simulink model "hcu_main_ADASwEPS"  (Simulink 8.2)
settings: Solver=FixedStepDiscrete  StartTime=0.0  StopTime=inf  FixedStep=0.001  RelTol=1e-3
PostLoadFcn:
  | , if any(exist('dsrtsu_mdlpostloadfcn', 'file') == [2, 3, 6]), try dsrtsu_mdlpostloadfcn('Execute', bdroot); catch fprintf('Error in PostLoadFcn (dsrtsu_mdlpostloadfcn) for model "%s":\n %s\n', bdroot, lasterr); end, end,
values from neighbouring files (symbols this model uses):
  C_TASK_1MS_S = (	C_TICK_TIME_S       )    [hcu_local_hdr.m]    (also in temp_ovrd_values.m = double(	0.001                  ))
  C_TICK_TIME_S = single(	0.005	    	)    [hcu_local_hdr.m]
  ENUM_EPSLFCSTATUS_ACTIVE = uint8(  2  )    [hcu_local_hdr.m]
  ENUM_EPSLFCSTATUS_TRANSITION = uint8(  3  )    [hcu_local_hdr.m]
  ENUM_EPSLKASTATUS_ACTIVE = uint8(  2  )    [hcu_local_hdr.m]
  ENUM_EPSMODEREQ_ANGLE = uint8(  1  )    [hcu_local_hdr.m]
  ENUM_EPSMODEREQ_INTERNAL = uint8(  0  )    [hcu_local_hdr.m]
  ENUM_EPSMODEREQ_TORQUE = uint8(  2  )    [hcu_local_hdr.m]
  ENUM_GEARPOSN_1ST = uint8(  1  )    [hcu_local_hdr.m]
  ENUM_GEARPOSN_2ND = uint8(  2  )    [hcu_local_hdr.m]
  ENUM_GEARPOSN_3RD = uint8(  3  )    [hcu_local_hdr.m]
  ENUM_GEARPOSN_4TH = uint8(  4  )    [hcu_local_hdr.m]
  ENUM_GEARPOSN_5TH = uint8(  5  )    [hcu_local_hdr.m]
  ENUM_GEARPOSN_6TH = uint8(  6  )    [hcu_local_hdr.m]
  ENUM_GEARPOSN_R = uint8(  7  )    [hcu_local_hdr.m]
  FALSE = boolean( 0 )    [hcu_local_hdr.m]
  TRUE = boolean( 1 )    [hcu_local_hdr.m]
undefined symbols (not defined in the file or in its folder): AISP_EPSCurrent_pct, AISP_TqASensorDelta_pct, AISP_TqBSensorDelta_pct, dHAL_IN, hal, INVALID_ABS1_TIMEOUT, INVALID_ABS2_TIMEOUT, INVALID_ABS3_TIMEOUT, INVALID_ABS4_TIMEOUT, INVALID_AC1_TIMEOUT, INVALID_ADASTORQ_REQ, INVALID_BCM1_TIMEOUT, INVALID_BCM2_TIMEOUT, INVALID_BOOSTER_VAC, INVALID_CSW1_TIMEOUT, INVALID_CUR_VEHDECE, INVALID_CURBRAKEDECE_REQ, INVALID_CURSTEERANG_REQ, INVALID_CURSTEERTQ_REQ, INVALID_ECM1_TIMEOUT, INVALID_ECM2_TIMEOUT, INVALID_ECM3_TIMEOUT, INVALID_ECM9_TIMEOUT, INVALID_ENG_TORQUE_FRICTIONAL, INVALID_ENG_TORQUE_INDICATED, INVALID_ENG_TORQUE_INDICATEDCOR, INVALID_ENG_TQ_MAX, INVALID_ENG_TQ_MIN, INVALID_EPAS2_TIMEOUT, INVALID_EPAS3_TIMEOUT, INVALID_EPB1_TIMEOUT, INVALID_EPS_BATTVOLT, INVALID_ESC_BATTVOLT, INVALID_GRADE, INVALID_HCU3_TIMEOUT, INVALID_HCU4_TIMEOUT, INVALID_HMI1_TIMEOUT, INVALID_HMI2_TIMEOUT, INVALID_LAT_ACC, INVALID_LONG_ACC, INVALID_MC_PRESSURE, INVALID_METER1_TIMEOUT, INVALID_METER3_TIMEOUT, INVALID_METER_VEHSPD, INVALID_ODO_METER, INVALID_OUTSIDE_TEMP, INVALID_PARKBRAKEBIND_STAT, INVALID_PEDALTQ_REQ, INVALID_SAS1_TIMEOUT, INVALID_SAS_ANGLE, INVALID_SHIFTER_POSN, INVALID_TCM1_TIMEOUT, INVALID_TCM2_TIMEOUT, INVALID_VCU1_TIMEOUT, INVALID_VCU2_TIMEOUT, INVALID_VEH_CRASH, INVALID_VEH_SPD, INVALID_WHEEL_SPD, INVALID_YAW_RATE, KHAL_MssgIdObj1_num ... (+8)
libraries: simulink x147, hcu_lib x38, rti1401lib_dio_type3 x4, rtimmsu_dsrtlib x3, app x1, rtiethernetudplib x1, rti1401lib_adc_type4 x1, rti1401lib_dac_type3 x1, inp x1, lidr x1, outp x1
(part 9 of 15)

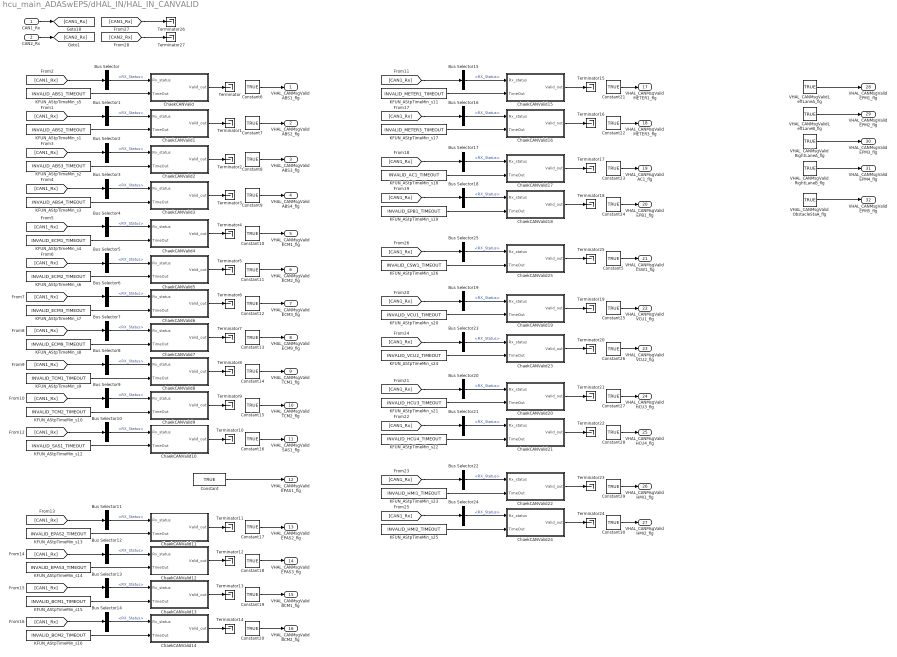
== system hcu_main_ADASwEPS/dHAL_IN/HAL_IN_CANVALID ==
  CAN1_Rx : Inport
  CAN2_Rx : Inport  Port=2
  Bus Selector : BusSelector  OutputSignals=ABS1.RX_Status
  Bus Selector1 : BusSelector  OutputSignals=ABS2.RX_Status
  Bus Selector10 : BusSelector  OutputSignals=SAS1.RX_Status
  Bus Selector11 : BusSelector  OutputSignals=EPAS2.RX_Status
  Bus Selector12 : BusSelector  OutputSignals=EPAS3.RX_Status
  Bus Selector13 : BusSelector  OutputSignals=BCM1.RX_Status
  Bus Selector14 : BusSelector  OutputSignals=BCM2.RX_Status
  Bus Selector15 : BusSelector  OutputSignals=Meter1.RX_Status
  Bus Selector16 : BusSelector  OutputSignals=Meter3.RX_Status
  Bus Selector17 : BusSelector  OutputSignals=AC1.RX_Status
  Bus Selector18 : BusSelector  OutputSignals=EPB1.RX_Status
  Bus Selector19 : BusSelector  OutputSignals=VCU1.RX_Status
  Bus Selector2 : BusSelector  OutputSignals=ABS3.RX_Status
  Bus Selector20 : BusSelector  OutputSignals=HCU3.RX_Status
  Bus Selector21 : BusSelector  OutputSignals=HCU4.RX_Status
  Bus Selector22 : BusSelector  OutputSignals=HMI1.RX_Status
  Bus Selector23 : BusSelector  OutputSignals=VCU2.RX_Status
  Bus Selector24 : BusSelector  OutputSignals=HMI2.RX_Status
  Bus Selector25 : BusSelector  OutputSignals=VCU1.RX_Status
  Bus Selector3 : BusSelector  OutputSignals=ABS4.RX_Status
  Bus Selector4 : BusSelector  OutputSignals=ECM1.RX_Status
  Bus Selector5 : BusSelector  OutputSignals=ECM2.RX_Status
  Bus Selector6 : BusSelector  OutputSignals=ECM3.RX_Status
  Bus Selector7 : BusSelector  OutputSignals=ECM9.RX_Status
  Bus Selector8 : BusSelector  OutputSignals=TCM1.RX_Status
  Bus Selector9 : BusSelector  OutputSignals=TCM2.RX_Status
  ChaekCANValid : Subsystem
  ChaekCANValid1 : Subsystem
  ChaekCANValid10 : Subsystem
  ChaekCANValid11 : Subsystem
  ChaekCANValid12 : Subsystem
  ChaekCANValid13 : Subsystem
  ChaekCANValid14 : Subsystem
  ChaekCANValid15 : Subsystem
  ChaekCANValid16 : Subsystem
  ChaekCANValid17 : Subsystem
  ChaekCANValid18 : Subsystem
  ChaekCANValid19 : Subsystem
  ChaekCANValid2 : Subsystem
  ChaekCANValid20 : Subsystem
  ChaekCANValid21 : Subsystem
  ChaekCANValid22 : Subsystem
  ChaekCANValid23 : Subsystem
  ChaekCANValid24 : Subsystem
  ChaekCANValid25 : Subsystem
  ChaekCANValid3 : Subsystem
  ChaekCANValid4 : Subsystem
  ChaekCANValid5 : Subsystem
  ChaekCANValid6 : Subsystem
  ChaekCANValid7 : Subsystem
  ChaekCANValid8 : Subsystem
  ChaekCANValid9 : Subsystem
  Constant{,5..30} (27 alike) : Constant  Value=TRUE
  KFUN_AStpTimeMin_s1 : Constant  Value=INVALID_ABS2_TIMEOUT
  KFUN_AStpTimeMin_s10 : Constant  Value=INVALID_TCM2_TIMEOUT
  KFUN_AStpTimeMin_s11 : Constant  Value=INVALID_METER1_TIMEOUT
  KFUN_AStpTimeMin_s12 : Constant  Value=INVALID_SAS1_TIMEOUT
  KFUN_AStpTimeMin_s13 : Constant  Value=INVALID_EPAS2_TIMEOUT
  KFUN_AStpTimeMin_s14 : Constant  Value=INVALID_EPAS3_TIMEOUT
  KFUN_AStpTimeMin_s15 : Constant  Value=INVALID_BCM1_TIMEOUT
  KFUN_AStpTimeMin_s16 : Constant  Value=INVALID_BCM2_TIMEOUT
  KFUN_AStpTimeMin_s17 : Constant  Value=INVALID_METER3_TIMEOUT
  KFUN_AStpTimeMin_s18 : Constant  Value=INVALID_AC1_TIMEOUT
  KFUN_AStpTimeMin_s19 : Constant  Value=INVALID_EPB1_TIMEOUT
  KFUN_AStpTimeMin_s2 : Constant  Value=INVALID_ABS3_TIMEOUT
  KFUN_AStpTimeMin_s20 : Constant  Value=INVALID_VCU1_TIMEOUT
  KFUN_AStpTimeMin_s21 : Constant  Value=INVALID_HCU3_TIMEOUT
  KFUN_AStpTimeMin_s22 : Constant  Value=INVALID_HCU4_TIMEOUT
  KFUN_AStpTimeMin_s23 : Constant  Value=INVALID_HMI1_TIMEOUT  VectorParams1D=off
  KFUN_AStpTimeMin_s24 : Constant  Value=INVALID_VCU2_TIMEOUT
  KFUN_AStpTimeMin_s25 : Constant  Value=INVALID_HMI2_TIMEOUT  VectorParams1D=off
  KFUN_AStpTimeMin_s26 : Constant  Value=INVALID_CSW1_TIMEOUT
  KFUN_AStpTimeMin_s3 : Constant  Value=INVALID_ABS4_TIMEOUT
  KFUN_AStpTimeMin_s4 : Constant  Value=INVALID_ECM1_TIMEOUT
  KFUN_AStpTimeMin_s5 : Constant  Value=INVALID_ABS1_TIMEOUT
  KFUN_AStpTimeMin_s6 : Constant  Value=INVALID_ECM2_TIMEOUT
  KFUN_AStpTimeMin_s7 : Constant  Value=INVALID_ECM3_TIMEOUT
  KFUN_AStpTimeMin_s8 : Constant  Value=INVALID_ECM9_TIMEOUT
  KFUN_AStpTimeMin_s9 : Constant  Value=INVALID_TCM1_TIMEOUT
  Terminator{,1..27} (28 alike) : Terminator
  VHAL_CANMsgValidLeftLaneA_flg : Constant  Value=TRUE
  VHAL_CANMsgValidLeftLaneB_flg : Constant  Value=TRUE
  VHAL_CANMsgValidObstacleStaA_flg : Constant  Value=TRUE
  VHAL_CANMsgValidRightLaneA_flg : Constant  Value=TRUE
  VHAL_CANMsgValidRightLaneB_flg : Constant  Value=TRUE
  VHAL_CANMsgValidABS1_flg : Outport
  VHAL_CANMsgValidABS2_flg : Outport  Port=2
  VHAL_CANMsgValidABS3_flg : Outport  Port=3
  VHAL_CANMsgValidABS4_flg : Outport  Port=4
  VHAL_CANMsgValidECM1_flg : Outport  Port=5
  VHAL_CANMsgValidECM2_flg : Outport  Port=6
  VHAL_CANMsgValidECM3_flg : Outport  Port=7
  VHAL_CANMsgValidECM9_flg : Outport  Port=8
  VHAL_CANMsgValidTCM1_flg : Outport  Port=9
  VHAL_CANMsgValidTCM2_flg : Outport  Port=10
  VHAL_CANMsgValidSAS1_flg : Outport  Port=11
  VHAL_CANMsgValidEPAS1_flg : Outport  Port=12
  VHAL_CANMsgValidEPAS2_flg : Outport  Port=13
  VHAL_CANMsgValidEPAS3_flg : Outport  Port=14
  VHAL_CANMsgValidBCM1_flg : Outport  Port=15
  VHAL_CANMsgValidBCM2_flg : Outport  Port=16
  VHAL_CANMsgValidMETER1_flg : Outport  Port=17
  VHAL_CANMsgValidMETER3_flg : Outport  Port=18
  VHAL_CANMsgValidAC1_flg : Outport  Port=19
  VHAL_CANMsgValidEPB1_flg : Outport  Port=20
  VHAL_CANMsgValidCSW1_flg : Outport  Port=21
  VHAL_CANMsgValidVCU1_flg : Outport  Port=22
  VHAL_CANMsgValidVCU2_flg : Outport  Port=23
  VHAL_CANMsgValidHCU3_flg : Outport  Port=24
  VHAL_CANMsgValidHCU4_flg : Outport  Port=25
  VHAL_CANMsgValidHMI1_flg : Outport  Port=26
  VHAL_CANMsgValidHMI2_flg : Outport  Port=27
  VHAL_CANMsgValidEPM1_flg : Outport  Port=28
  VHAL_CANMsgValidEPM2_flg : Outport  Port=29
  VHAL_CANMsgValidEPM3_flg : Outport  Port=30
  VHAL_CANMsgValidEPM4_flg : Outport  Port=31
  VHAL_CANMsgValidEPM5_flg : Outport  Port=32
  wires:
  ChaekCANValid24/1(Valid_out) -> Terminator24/1
  Constant30/1 -> VHAL_CANMsgValidHMI2_flg/1
  ChaekCANValid22/1(Valid_out) -> Terminator23/1
  Constant29/1 -> VHAL_CANMsgValidHMI1_flg/1
  ChaekCANValid21/1(Valid_out) -> Terminator22/1
  Constant28/1 -> VHAL_CANMsgValidHCU4_flg/1
  ChaekCANValid20/1(Valid_out) -> Terminator21/1
  Constant27/1 -> VHAL_CANMsgValidHCU3_flg/1
  ChaekCANValid23/1(Valid_out) -> Terminator20/1
  Constant26/1 -> VHAL_CANMsgValidVCU2_flg/1
  ChaekCANValid19/1(Valid_out) -> Terminator19/1
  Constant25/1 -> VHAL_CANMsgValidVCU1_flg/1
  ChaekCANValid18/1(Valid_out) -> Terminator18/1
  Constant24/1 -> VHAL_CANMsgValidEPB1_flg/1
  ChaekCANValid17/1(Valid_out) -> Terminator17/1
  Constant23/1 -> VHAL_CANMsgValidAC1_flg/1
  ChaekCANValid16/1(Valid_out) -> Terminator16/1
  Constant22/1 -> VHAL_CANMsgValidMETER3_flg/1
  ChaekCANValid15/1(Valid_out) -> Terminator15/1
  Constant21/1 -> VHAL_CANMsgValidMETER1_flg/1
  ChaekCANValid14/1(Valid_out) -> Terminator14/1
  Constant20/1 -> VHAL_CANMsgValidBCM2_flg/1
  ChaekCANValid13/1(Valid_out) -> Terminator13/1
  Constant19/1 -> VHAL_CANMsgValidBCM1_flg/1
  ChaekCANValid12/1(Valid_out) -> Terminator12/1
  Constant18/1 -> VHAL_CANMsgValidEPAS3_flg/1
  ChaekCANValid11/1(Valid_out) -> Terminator11/1
  Constant17/1 -> VHAL_CANMsgValidEPAS2_flg/1
  ChaekCANValid10/1(Valid_out) -> Terminator10/1
  Constant16/1 -> VHAL_CANMsgValidSAS1_flg/1
  ChaekCANValid9/1(Valid_out) -> Terminator9/1
  Constant15/1 -> VHAL_CANMsgValidTCM2_flg/1
  ChaekCANValid8/1(Valid_out) -> Terminator8/1
  Constant14/1 -> VHAL_CANMsgValidTCM1_flg/1
  ChaekCANValid7/1(Valid_out) -> Terminator7/1
  Constant13/1 -> VHAL_CANMsgValidECM9_flg/1
  Constant12/1 -> VHAL_CANMsgValidECM3_flg/1
  ChaekCANValid6/1(Valid_out) -> Terminator6/1
  ChaekCANValid5/1(Valid_out) -> Terminator5/1
  Constant11/1 -> VHAL_CANMsgValidECM2_flg/1
  ChaekCANValid4/1(Valid_out) -> Terminator4/1
  Constant10/1 -> VHAL_CANMsgValidECM1_flg/1
  ChaekCANValid3/1(Valid_out) -> Terminator3/1
  Constant9/1 -> VHAL_CANMsgValidABS4_flg/1
  ChaekCANValid2/1(Valid_out) -> Terminator2/1
  Constant8/1 -> VHAL_CANMsgValidABS3_flg/1
  Constant7/1 -> VHAL_CANMsgValidABS2_flg/1
  ChaekCANValid1/1(Valid_out) -> Terminator1/1
  Constant6/1 -> VHAL_CANMsgValidABS1_flg/1
  ChaekCANValid/1(Valid_out) -> Terminator/1
  KFUN_AStpTimeMin_s25/1 -> ChaekCANValid24/2(TimeOut)
  Bus Selector24/1 -> ChaekCANValid24/1(Rx_status)  "<RX_Status>"
  [CAN1_Rx] -> Bus Selector24/1
  CAN2_Rx/1 -> [CAN2_Rx]
  KFUN_AStpTimeMin_s24/1 -> ChaekCANValid23/2(TimeOut)
  Bus Selector23/1 -> ChaekCANValid23/1(Rx_status)  "<RX_Status>"
  [CAN1_Rx] -> Bus Selector23/1
  KFUN_AStpTimeMin_s23/1 -> ChaekCANValid22/2(TimeOut)
  Bus Selector22/1 -> ChaekCANValid22/1(Rx_status)  "<RX_Status>"
  [CAN1_Rx] -> Bus Selector22/1
  KFUN_AStpTimeMin_s22/1 -> ChaekCANValid21/2(TimeOut)
  Bus Selector21/1 -> ChaekCANValid21/1(Rx_status)  "<RX_Status>"
  [CAN1_Rx] -> Bus Selector21/1
  KFUN_AStpTimeMin_s21/1 -> ChaekCANValid20/2(TimeOut)
  Bus Selector20/1 -> ChaekCANValid20/1(Rx_status)  "<RX_Status>"
  [CAN1_Rx] -> Bus Selector20/1
  KFUN_AStpTimeMin_s20/1 -> ChaekCANValid19/2(TimeOut)
  Bus Selector19/1 -> ChaekCANValid19/1(Rx_status)  "<RX_Status>"
  [CAN1_Rx] -> Bus Selector19/1
  KFUN_AStpTimeMin_s19/1 -> ChaekCANValid18/2(TimeOut)
  Bus Selector18/1 -> ChaekCANValid18/1(Rx_status)  "<RX_Status>"
  [CAN1_Rx] -> Bus Selector18/1
  KFUN_AStpTimeMin_s18/1 -> ChaekCANValid17/2(TimeOut)
  Bus Selector17/1 -> ChaekCANValid17/1(Rx_status)  "<RX_Status>"
  [CAN1_Rx] -> Bus Selector17/1
  KFUN_AStpTimeMin_s17/1 -> ChaekCANValid16/2(TimeOut)
  Bus Selector16/1 -> ChaekCANValid16/1(Rx_status)  "<RX_Status>"
  [CAN1_Rx] -> Bus Selector16/1
  KFUN_AStpTimeMin_s11/1 -> ChaekCANValid15/2(TimeOut)
  Bus Selector15/1 -> ChaekCANValid15/1(Rx_status)  "<RX_Status>"
  [CAN1_Rx] -> Bus Selector15/1
  KFUN_AStpTimeMin_s16/1 -> ChaekCANValid14/2(TimeOut)
  Bus Selector14/1 -> ChaekCANValid14/1(Rx_status)  "<RX_Status>"
  [CAN1_Rx] -> Bus Selector14/1
  KFUN_AStpTimeMin_s15/1 -> ChaekCANValid13/2(TimeOut)
  Bus Selector13/1 -> ChaekCANValid13/1(Rx_status)  "<RX_Status>"
  [CAN1_Rx] -> Bus Selector13/1
  KFUN_AStpTimeMin_s14/1 -> ChaekCANValid12/2(TimeOut)
  Bus Selector12/1 -> ChaekCANValid12/1(Rx_status)  "<RX_Status>"
  [CAN1_Rx] -> Bus Selector12/1
  KFUN_AStpTimeMin_s13/1 -> ChaekCANValid11/2(TimeOut)
  Bus Selector11/1 -> ChaekCANValid11/1(Rx_status)  "<RX_Status>"
  [CAN1_Rx] -> Bus Selector11/1
  KFUN_AStpTimeMin_s12/1 -> ChaekCANValid10/2(TimeOut)
  Bus Selector10/1 -> ChaekCANValid10/1(Rx_status)  "<RX_Status>"
  [CAN1_Rx] -> Bus Selector10/1
  KFUN_AStpTimeMin_s10/1 -> ChaekCANValid9/2(TimeOut)
  Bus Selector9/1 -> ChaekCANValid9/1(Rx_status)  "<RX_Status>"
  [CAN1_Rx] -> Bus Selector9/1
  KFUN_AStpTimeMin_s9/1 -> ChaekCANValid8/2(TimeOut)
  Bus Selector8/1 -> ChaekCANValid8/1(Rx_status)  "<RX_Status>"
  [CAN1_Rx] -> Bus Selector8/1
  KFUN_AStpTimeMin_s8/1 -> ChaekCANValid7/2(TimeOut)
  Bus Selector7/1 -> ChaekCANValid7/1(Rx_status)  "<RX_Status>"
  [CAN1_Rx] -> Bus Selector7/1
  KFUN_AStpTimeMin_s7/1 -> ChaekCANValid6/2(TimeOut)
  Bus Selector6/1 -> ChaekCANValid6/1(Rx_status)  "<RX_Status>"
  [CAN1_Rx] -> Bus Selector6/1
  KFUN_AStpTimeMin_s6/1 -> ChaekCANValid5/2(TimeOut)
  Bus Selector5/1 -> ChaekCANValid5/1(Rx_status)  "<RX_Status>"
  [CAN1_Rx] -> Bus Selector5/1
  KFUN_AStpTimeMin_s4/1 -> ChaekCANValid4/2(TimeOut)
  Bus Selector4/1 -> ChaekCANValid4/1(Rx_status)  "<RX_Status>"
  [CAN1_Rx] -> Bus Selector4/1
  KFUN_AStpTimeMin_s3/1 -> ChaekCANValid3/2(TimeOut)
  Bus Selector3/1 -> ChaekCANValid3/1(Rx_status)  "<RX_Status>"
  [CAN1_Rx] -> Bus Selector3/1
  KFUN_AStpTimeMin_s2/1 -> ChaekCANValid2/2(TimeOut)
  Bus Selector2/1 -> ChaekCANValid2/1(Rx_status)  "<RX_Status>"
  [CAN1_Rx] -> Bus Selector2/1
  KFUN_AStpTimeMin_s1/1 -> ChaekCANValid1/2(TimeOut)
  Bus Selector1/1 -> ChaekCANValid1/1(Rx_status)  "<RX_Status>"
  [CAN1_Rx] -> Bus Selector1/1
  CAN1_Rx/1 -> [CAN1_Rx]
  KFUN_AStpTimeMin_s5/1 -> ChaekCANValid/2(TimeOut)
  Bus Selector/1 -> ChaekCANValid/1(Rx_status)  "<RX_Status>"
  [CAN1_Rx] -> Bus Selector/1
  VHAL_CANMsgValidLeftLaneA_flg/1 -> VHAL_CANMsgValidEPM1_flg/1
  VHAL_CANMsgValidLeftLaneB_flg/1 -> VHAL_CANMsgValidEPM2_flg/1
  VHAL_CANMsgValidRightLaneA_flg/1 -> VHAL_CANMsgValidEPM3_flg/1
  VHAL_CANMsgValidRightLaneB_flg/1 -> VHAL_CANMsgValidEPM4_flg/1
  Constant/1 -> VHAL_CANMsgValidEPAS1_flg/1
  ChaekCANValid25/1(Valid_out) -> Terminator25/1
  Constant5/1 -> VHAL_CANMsgValidCSW1_flg/1
  KFUN_AStpTimeMin_s26/1 -> ChaekCANValid25/2(TimeOut)
  Bus Selector25/1 -> ChaekCANValid25/1(Rx_status)  "<RX_Status>"
  [CAN1_Rx] -> Bus Selector25/1
  VHAL_CANMsgValidObstacleStaA_flg/1 -> VHAL_CANMsgValidEPM5_flg/1
  [CAN1_Rx] -> Terminator26/1
  [CAN2_Rx] -> Terminator27/1

== system hcu_main_ADASwEPS/dHAL_IN/HAL_IN_CSW ==
  CAN1_Rx : Inport
  BO__1040_CSW1__8_CSW : Subsystem
  VHAL_RearFogSwOn_flg : Outport
  VHAL_HighBeamSwOn_flg : Outport  Port=2
  wires:
  [CAN1_Rx] -> BO__1040_CSW1__8_CSW/1(CAN1_Rx)
  CAN1_Rx/1 -> [CAN1_Rx]
  BO__1040_CSW1__8_CSW/1(CSW_RFogLpSw_Sta) -> VHAL_RearFogSwOn_flg/1
  BO__1040_CSW1__8_CSW/2(CSW_DimSw_Sta) -> VHAL_HighBeamSwOn_flg/1

== system hcu_main_ADASwEPS/dHAL_IN/HAL_IN_EPB ==
  CAN1_Rx : Inport
  BO__928_EPB1__8_EPB : Subsystem
  KFUN_AStpTimeMin_s3 : Constant  Value=INVALID_PARKBRAKEBIND_STAT
  Relational Operator3 : RelationalOperator  Operator===  OutDataTypeStr=boolean
  VHAL_ParkBrakeBindSta_enum : Outport
  VHAL_ParkBrakeBindStaInvalid_flg : Outport  Port=2
  wires:
  KFUN_AStpTimeMin_s3/1 -> Relational Operator3/2
  Relational Operator3/1 -> VHAL_ParkBrakeBindStaInvalid_flg/1
  BO__928_EPB1__8_EPB/1(PB_BrakeBinStat) -> Relational Operator3/1, VHAL_ParkBrakeBindSta_enum/1
  CAN1_Rx/1 -> [CAN1_Rx]
  [CAN1_Rx] -> BO__928_EPB1__8_EPB/1(CAN1_Rx)

== system hcu_main_ADASwEPS/dHAL_IN/HAL_IN_EPM ==
  CAN2_Rx : Inport
  BO__1347_LKA_Left_Lane_A__8_EPM : Subsystem
  BO__1347_LKA_Left_Lane_B__8_EPM : Subsystem
  BO__1347_LKA_Right_Lane_A__8_EPM : Subsystem
  BO__1347_LKA_Right_Lane_B__8_EPM : Subsystem
  BO__1848_ObstacleStatusA__8_EPM : Subsystem
  VHAL_LaneQualityL_enum : Outport
  VHAL_LaneQualityR_enum : Outport  Port=2
  VHAL_LaneC0L_m : Outport  Port=3
  VHAL_LaneC1L_rad : Outport  Port=4
  VHAL_LaneC2L_rat : Outport  Port=5
  VHAL_LaneC3L_rat : Outport  Port=6
  VHAL_LaneC0R_m : Outport  Port=7
  VHAL_LaneC1R_rad : Outport  Port=8
  VHAL_LaneC2R_rat : Outport  Port=9
  VHAL_LaneC3R_rat : Outport  Port=10
  VHAL_LaneTypeL_enum : Outport  Port=11
  VHAL_LaneTypeR_enum : Outport  Port=12
  VHAL_LaneMrkWidL_m : Outport  Port=13
  VHAL_LaneMrkWidR_m : Outport  Port=14
  VHAL_ViewRangeStartL_m : Outport  Port=15
  VHAL_ViewRangeEndL_m : Outport  Port=16
  VHAL_ViewRangeStartR_m : Outport  Port=17
  VHAL_ViewRangeEndR_m : Outport  Port=18
  VHAL_LaneCrosL_flg : Outport  Port=19
  VHAL_LaneCrosR_flg : Outport  Port=20
  VHAL_LaneMrkClrL_enum : Outport  Port=21
  VHAL_LaneMrkClrR_enum : Outport  Port=22
  VHAL_TLCL_s : Outport  Port=23
  VHAL_TLCR_s : Outport  Port=24
  VHAL_CamNofObjects_num : Outport  Port=25
  VHAL_CamGoDecision_enum : Outport  Port=26
  VHAL_CloseCarDetected_flg : Outport  Port=27
  VHAL_RightCarCutIn_flg : Outport  Port=28
  VHAL_LeftCarCutIn_flg : Outport  Port=29
  VHAL_CamFSImpairedVD_flg : Outport  Port=30
  VHAL_CamFSLowSun_flg : Outport  Port=31
  VHAL_CamFSBlurImage_flg : Outport  Port=32
  VHAL_CamFSSmearImage_flg : Outport  Port=33
  VHAL_CamFSPartialBlockage_flg : Outport  Port=34
  VHAL_CamFSFullBlockage_flg : Outport  Port=35
  VHAL_CamFSSplashes_flg : Outport  Port=36
  VHAL_CamFSOutofCal_flg : Outport  Port=37
  VHAL_CamFSCalMisalign_flg : Outport  Port=38
  VHAL_CamFSSmearedspots_flg : Outport  Port=39
  VHAL_CamFSSpotHalosFrozen_flg : Outport  Port=40
  VHAL_CamFSFoggySpots_flg : Outport  Port=41
  VHAL_CamFSSunRay_flg : Outport  Port=42
  wires:
  CAN2_Rx/1 -> [CAN2_Rx]
  [CAN2_Rx] -> BO__1347_LKA_Left_Lane_A__8_EPM/1(CAN2_Rx)
  [CAN2_Rx] -> BO__1347_LKA_Left_Lane_B__8_EPM/1(CAN2_Rx)
  [CAN2_Rx] -> BO__1347_LKA_Right_Lane_A__8_EPM/1(CAN2_Rx)
  [CAN2_Rx] -> BO__1347_LKA_Right_Lane_B__8_EPM/1(CAN2_Rx)
  BO__1347_LKA_Left_Lane_A__8_EPM/5(VHAL_LaneC3L_rat) -> VHAL_LaneC3L_rat/1
  BO__1347_LKA_Left_Lane_A__8_EPM/2(VHAL_LaneQualityL_enum) -> VHAL_LaneQualityL_enum/1
  BO__1347_LKA_Left_Lane_A__8_EPM/6(VHAL_LaneMrkWidL_m) -> VHAL_LaneMrkWidL_m/1
  BO__1347_LKA_Left_Lane_A__8_EPM/4(VHAL_LaneC2L_rat) -> VHAL_LaneC2L_rat/1
  BO__1347_LKA_Left_Lane_A__8_EPM/3(VHAL_LaneC0L_m) -> VHAL_LaneC0L_m/1
  BO__1347_LKA_Left_Lane_A__8_EPM/1(VHAL_LaneTypeL_enum) -> VHAL_LaneTypeL_enum/1
  BO__1347_LKA_Left_Lane_B__8_EPM/3(VHAL_ViewRangeEndL_m) -> VHAL_ViewRangeEndL_m/1
  BO__1347_LKA_Left_Lane_B__8_EPM/5(VHAL_LaneMrkClrL_enum) -> VHAL_LaneMrkClrL_enum/1
  BO__1347_LKA_Left_Lane_B__8_EPM/1(VHAL_LaneC1L_rad) -> VHAL_LaneC1L_rad/1
  BO__1347_LKA_Left_Lane_B__8_EPM/4(VHAL_LaneCrossingL_flg) -> VHAL_LaneCrosL_flg/1
  BO__1347_LKA_Left_Lane_B__8_EPM/2(VHAL_ViewRangeStartL_m) -> VHAL_ViewRangeStartL_m/1
  BO__1347_LKA_Left_Lane_B__8_EPM/6(VHAL_TLCL_s) -> VHAL_TLCL_s/1
  BO__1347_LKA_Right_Lane_A__8_EPM/3(VHAL_LaneC0R_m) -> VHAL_LaneC0R_m/1
  BO__1347_LKA_Right_Lane_A__8_EPM/5(VHAL_LaneC3R_rat) -> VHAL_LaneC3R_rat/1
  BO__1347_LKA_Right_Lane_A__8_EPM/1(VHAL_LaneTypeR_enum) -> VHAL_LaneTypeR_enum/1
  BO__1347_LKA_Right_Lane_A__8_EPM/4(VHAL_LaneC2R_rat) -> VHAL_LaneC2R_rat/1
  BO__1347_LKA_Right_Lane_A__8_EPM/2(VHAL_LaneQualityR_enum) -> VHAL_LaneQualityR_enum/1
  BO__1347_LKA_Right_Lane_A__8_EPM/6(VHAL_LaneMrkWidR_m) -> VHAL_LaneMrkWidR_m/1
  BO__1347_LKA_Right_Lane_B__8_EPM/3(VHAL_ViewRangeEndR_m) -> VHAL_ViewRangeEndR_m/1
  BO__1347_LKA_Right_Lane_B__8_EPM/2(VHAL_ViewRangeStartR_m) -> VHAL_ViewRangeStartR_m/1
  BO__1347_LKA_Right_Lane_B__8_EPM/4(VHAL_LaneCrossingR_flg) -> VHAL_LaneCrosR_flg/1
  BO__1347_LKA_Right_Lane_B__8_EPM/1(VHAL_LaneC1R_rad) -> VHAL_LaneC1R_rad/1
  BO__1347_LKA_Right_Lane_B__8_EPM/5(VHAL_LaneMrkClrR_enum) -> VHAL_LaneMrkClrR_enum/1
  BO__1347_LKA_Right_Lane_B__8_EPM/6(VHAL_TLCR_s) -> VHAL_TLCR_s/1
  [CAN2_Rx] -> BO__1848_ObstacleStatusA__8_EPM/1(CAN2_Rx)
  BO__1848_ObstacleStatusA__8_EPM/1(VHAL_CamNofObjects_num) -> VHAL_CamNofObjects_num/1
  BO__1848_ObstacleStatusA__8_EPM/2(VHAL_CamGoDecision_enum) -> VHAL_CamGoDecision_enum/1
  BO__1848_ObstacleStatusA__8_EPM/3(VHAL_CloseCarDetected_flg) -> VHAL_CloseCarDetected_flg/1
  BO__1848_ObstacleStatusA__8_EPM/4(VHAL_RightCarCutIn_flg) -> VHAL_RightCarCutIn_flg/1
  BO__1848_ObstacleStatusA__8_EPM/5(VHAL_LeftCarCutIn_flg) -> VHAL_LeftCarCutIn_flg/1
  BO__1848_ObstacleStatusA__8_EPM/6(VHAL_CamFSImpairedVD_flg) -> VHAL_CamFSImpairedVD_flg/1
  BO__1848_ObstacleStatusA__8_EPM/7(VHAL_CamFSLowSun_flg) -> VHAL_CamFSLowSun_flg/1
  BO__1848_ObstacleStatusA__8_EPM/8(VHAL_CamFSBlurImage_flg) -> VHAL_CamFSBlurImage_flg/1
  BO__1848_ObstacleStatusA__8_EPM/9(VHAL_CamFSSmearImage_flg) -> VHAL_CamFSSmearImage_flg/1
  BO__1848_ObstacleStatusA__8_EPM/10(VHAL_CamFSPartialBlockage_flg) -> VHAL_CamFSPartialBlockage_flg/1
  BO__1848_ObstacleStatusA__8_EPM/11(VHAL_CamFSFullBlockage_flg) -> VHAL_CamFSFullBlockage_flg/1
  BO__1848_ObstacleStatusA__8_EPM/12(VHAL_CamFSSplashes_flg) -> VHAL_CamFSSplashes_flg/1
  BO__1848_ObstacleStatusA__8_EPM/13(VHAL_CamFSOutofCal_flg) -> VHAL_CamFSOutofCal_flg/1
  BO__1848_ObstacleStatusA__8_EPM/14(VHAL_CamFSCalMisalign_flg) -> VHAL_CamFSCalMisalign_flg/1
  BO__1848_ObstacleStatusA__8_EPM/15(VHAL_CamFSSmearedspots_flg) -> VHAL_CamFSSmearedspots_flg/1
  BO__1848_ObstacleStatusA__8_EPM/16(VHAL_CamFSSpotHalosFrozen_flg) -> VHAL_CamFSSpotHalosFrozen_flg/1
  BO__1848_ObstacleStatusA__8_EPM/17(VHAL_CamFSFoggySpots_flg) -> VHAL_CamFSFoggySpots_flg/1
  BO__1848_ObstacleStatusA__8_EPM/18(VHAL_CamFSSunRay_flg) -> VHAL_CamFSSunRay_flg/1

== system hcu_main_ADASwEPS/dHAL_IN/HAL_IN_HMI ==
  CAN1_Rx : Inport
  BO__1347_HMI1__8_HMI : Subsystem
  Detect Change{,1..11} (12 alike) : simulink/Logic and Bit Operations/Detect Change  vinit=0  InputProcessing=Inherited  OutDataTypeStr=boolean
  VHAL_AEBEnableH_flg : Outport
  VHAL_FCWEnableH_flg : Outport  Port=2
  VHAL_CSCEnableH_flg : Outport  Port=3
  VHAL_LKAEnableH_flg : Outport  Port=4
  VHAL_MAPAEnableH_flg : Outport  Port=5
  VHAL_LCSEnableH_flg : Outport  Port=6
  VHAL_LFCPilotOnH_flg : Outport  Port=7
  VHAL_LFCPilotCancelH_flg : Outport  Port=8
  VHAL_ACCOnH_flg : Outport  Port=9
  VHAL_ACCCancelH_flg : Outport  Port=10
  VHAL_ACCResSpdIncH_flg : Outport  Port=11
  VHAL_ACCSetSpdDecH_flg : Outport  Port=12
  VHAL_ACCSpdIncH_flg : Outport  Port=13
  VHAL_ACCSpdDecH_flg : Outport  Port=14
  VHAL_ACCTimeGapIncH_flg : Outport  Port=15
  VHAL_ACCTimeGapDecH_flg : Outport  Port=16
  VHAL_IGSAOnH_flg : Outport  Port=17
  VHAL_IGSAResSpdIncH_flg : Outport  Port=18
  VHAL_IGSASetSpdDecH_flg : Outport  Port=19
  VHAL_IGSASwitchModeH_flg : Outport  Port=20
  VHAL_FCWWarningModeH_enum : Outport  Port=21
  VHAL_DefMaxACCSetSpeed_kph : Outport  Port=22
  wires:
  BO__1347_HMI1__8_HMI/1(ACCCancel) -> Detect Change/1
  BO__1347_HMI1__8_HMI/2(ACCOn) -> VHAL_ACCOnH_flg/1
  BO__1347_HMI1__8_HMI/3(ACCRes_SpdInc) -> Detect Change1/1
  BO__1347_HMI1__8_HMI/4(ACCSet_SpdDec) -> Detect Change2/1
  BO__1347_HMI1__8_HMI/7(ACCTimeGapDec) -> Detect Change5/1
  BO__1347_HMI1__8_HMI/8(ACCTimeGapInc) -> Detect Change6/1
  BO__1347_HMI1__8_HMI/9(AEBEnable) -> VHAL_AEBEnableH_flg/1
  BO__1347_HMI1__8_HMI/10(CSCEnable) -> VHAL_CSCEnableH_flg/1
  BO__1347_HMI1__8_HMI/11(FCWEnable) -> VHAL_FCWEnableH_flg/1
  BO__1347_HMI1__8_HMI/12(IGSAOn) -> VHAL_IGSAOnH_flg/1
  BO__1347_HMI1__8_HMI/13(IGSARes_SpdInc) -> Detect Change7/1
  BO__1347_HMI1__8_HMI/14(IGSASet_SpdDec) -> Detect Change8/1
  BO__1347_HMI1__8_HMI/15(IGSASwitchMode) -> Detect Change9/1
  BO__1347_HMI1__8_HMI/16(LCSEnable) -> VHAL_LCSEnableH_flg/1
  BO__1347_HMI1__8_HMI/17(LFC_PilotCancel) -> Detect Change10/1
  BO__1347_HMI1__8_HMI/18(LFC_PilotOn) -> Detect Change11/1
  BO__1347_HMI1__8_HMI/19(LKAEnable) -> VHAL_LKAEnableH_flg/1
  BO__1347_HMI1__8_HMI/20(MAPAEnable) -> VHAL_MAPAEnableH_flg/1
  CAN1_Rx/1 -> [CAN1_Rx]
  [CAN1_Rx] -> BO__1347_HMI1__8_HMI/1(CAN1_Rx)
  Detect Change/1 -> VHAL_ACCCancelH_flg/1
  Detect Change1/1 -> VHAL_ACCResSpdIncH_flg/1
  Detect Change2/1 -> VHAL_ACCSetSpdDecH_flg/1
  BO__1347_HMI1__8_HMI/5(ACCSpeedDec) -> Detect Change3/1
  BO__1347_HMI1__8_HMI/6(ACCSpeedInc) -> Detect Change4/1
  Detect Change5/1 -> VHAL_ACCTimeGapDecH_flg/1
  Detect Change6/1 -> VHAL_ACCTimeGapIncH_flg/1
  Detect Change7/1 -> VHAL_IGSAResSpdIncH_flg/1
  Detect Change8/1 -> VHAL_IGSASetSpdDecH_flg/1
  BO__1347_HMI1__8_HMI/21(FCWWarningMode) -> VHAL_FCWWarningModeH_enum/1
  BO__1347_HMI1__8_HMI/22(DefMaxACCSetSpeed) -> VHAL_DefMaxACCSetSpeed_kph/1
  Detect Change3/1 -> VHAL_ACCSpdDecH_flg/1
  Detect Change4/1 -> VHAL_ACCSpdIncH_flg/1
  Detect Change9/1 -> VHAL_IGSASwitchModeH_flg/1
  Detect Change10/1 -> VHAL_LFCPilotCancelH_flg/1
  Detect Change11/1 -> VHAL_LFCPilotOnH_flg/1

== system hcu_main_ADASwEPS/dHAL_IN/HAL_IN_RadObjDecoder ==
  CAN2_Rx : Inport
  Bus Selector : BusSelector  OutputSignals=RTICANMMCaptureMessage_1.Status,RTICANMMCaptureMessage_2.Status,RTICANMMCaptureMessage_3.Status,RTICANMMCaptureMessage_4.Status,RTICANMMCaptureMessage_5.Status,RTICANMMCaptureMessage_6.Status,RTICANMMCaptureMessage_7.Status,RTICANMMCaptureMessage_8.Status,RTICANMMCaptureMessage_9.Status,RTICANMMCaptureMessage_10.Status,RTICANMMCaptureMessage_11.Status,RTICANMMCaptureMessage_12.Status,RTICANMMCaptureMessage_13.Status,RTICANMMCaptureMessage_14.Status,RTICANMMCaptureMessage_15.Status,RTICANMMCaptureMessage_16.Status,RTICANMMCaptureMessage_17.Status,RTICANMMCaptureMessage_18.Status,RTICANMMCaptureMessage_19.Status,RTICANMMCaptureMessage_20.Status,RTICANMMCaptureMessage_21.Status,RTICANMMCaptureMessage_22.Status,RTICANMMCaptureMessage_23.Status,RTICANMMCaptureMessage_24.Status,RTICANMMCaptureMessage_25.Status
  Bus Selector1 : BusSelector  OutputSignals=RTICANMMCaptureMessage_1,RTICANMMCaptureMessage_2,RTICANMMCaptureMessage_3,RTICANMMCaptureMessage_4,RTICANMMCaptureMessage_5,RTICANMMCaptureMessage_6,RTICANMMCaptureMessage_7,RTICANMMCaptureMessage_8,RTICANMMCaptureMessage_9,RTICANMMCaptureMessage_10,RTICANMMCaptureMessage_11,RTICANMMCaptureMessage_12,RTICANMMCaptureMessage_13,RTICANMMCaptureMessage_14,RTICANMMCaptureMessage_15,RTICANMMCaptureMessage_16,RTICANMMCaptureMessage_17,RTICANMMCaptureMessage_18,RTICANMMCaptureMessage_19,RTICANMMCaptureMessage_20,RTICANMMCaptureMessage_21,RTICANMMCaptureMessage_22,RTICANMMCaptureMessage_23,RTICANMMCaptureMessage_24,RTICANMMCaptureMessage_25
  Bus Selector2 : BusSelector  OutputSignals=StatusFrame,Frames1,Frames2
  Ground : Ground
  N_of_CANData : Sum  Inputs=+++++++++++++++++++++++++
  RObj_Parser : Subsystem
  RObjectPackFrame : Subsystem  TreatAsAtomicUnit=on
  VHAL_RadNofObjects_num : Outport
  VHAL_MeasCounter_num : Outport  Port=2
  VHAL_SensorRxInvalid_enum : Outport  Port=3
  VHAL_SensorSupplyVoltage_V : Outport  Port=4
  VHAL_SensorDefective_enum : Outport  Port=5
  VHAL_SensorMisaligned_enum : Outport  Port=6
  VHAL_SensorSwitchedOff_enum : Outport  Port=7
  VHAL_SensorExternalDisturbed_enum : Outport  Port=8
  VHAL_SensorOutputReduced_enum : Outport  Port=9
  VHAL_LatDistToborderLeft_m : Outport  Port=10
  VHAL_LatDistToborderRight_m : Outport  Port=11
  VHAL_RadObjRolCountVect40_num : Outport  Port=12
  VHAL_RadObjIDVect40_num : Outport  Port=13
  VHAL_RadObjXDisplVect40_m : Outport  Port=14
  VHAL_RadObjVrelXVect40_mps : Outport  Port=15
  VHAL_RadObjAccelXVect40_mps2 : Outport  Port=16
  VHAL_RadObjYDisplVect40_m : Outport  Port=17
  VHAL_RadObjDynPropVect40_enum : Outport  Port=18
  VHAL_RadObjPExistVect40_enum : Outport  Port=19
  VHAL_RadObjMeasStatVect40_enum : Outport  Port=20
  VHAL_RadObjWidthVect40_m : Outport  Port=21
  VHAL_RadObjLengthVect40_m : Outport  Port=22
  VHAL_RadObjRCSVect40_num : Outport  Port=23
  VHAL_RadObjVrelYVect40_mps : Outport  Port=24
  VHAL_RadObjProbVect40_num : Outport  Port=25
  VHAL_RadWarningLevel_enum : Outport  Port=26
  VHAL_RadWarningObjID_num : Outport  Port=27
  wires:
  Ground/1 -> RObj_Parser/4(RObj_CollDetWarn)
  Bus Selector/1 -> N_of_CANData/1  "<Status>"
  Bus Selector/2 -> N_of_CANData/2  "<Status>"
  Bus Selector/3 -> N_of_CANData/3  "<Status>"
  Bus Selector/4 -> N_of_CANData/4  "<Status>"
  Bus Selector/5 -> N_of_CANData/5  "<Status>"
  Bus Selector/6 -> N_of_CANData/6  "<Status>"
  Bus Selector/7 -> N_of_CANData/7  "<Status>"
  Bus Selector/8 -> N_of_CANData/8  "<Status>"
  Bus Selector/9 -> N_of_CANData/9  "<Status>"
  Bus Selector/10 -> N_of_CANData/10  "<Status>"
  Bus Selector/11 -> N_of_CANData/11  "<Status>"
  Bus Selector/12 -> N_of_CANData/12  "<Status>"
  Bus Selector/13 -> N_of_CANData/13  "<Status>"
  Bus Selector/14 -> N_of_CANData/14  "<Status>"
  Bus Selector/15 -> N_of_CANData/15  "<Status>"
  Bus Selector/16 -> N_of_CANData/16  "<Status>"
  Bus Selector/17 -> N_of_CANData/17  "<Status>"
  Bus Selector/18 -> N_of_CANData/18  "<Status>"
  Bus Selector/19 -> N_of_CANData/19  "<Status>"
  Bus Selector/20 -> N_of_CANData/20  "<Status>"
  Bus Selector/21 -> N_of_CANData/21  "<Status>"
  Bus Selector/22 -> N_of_CANData/22  "<Status>"
  Bus Selector/23 -> N_of_CANData/23  "<Status>"
  Bus Selector/24 -> N_of_CANData/24  "<Status>"
  Bus Selector/25 -> N_of_CANData/25  "<Status>"
  N_of_CANData/1 -> RObjectPackFrame/1(CAN_Frames)
  Bus Selector1/4 -> RObjectPackFrame/5(CaptureMessage4)  "<RTICANMMCaptureMessage_4>"
  Bus Selector1/7 -> RObjectPackFrame/8(CaptureMessage7)  "<RTICANMMCaptureMessage_7>"
  Bus Selector1/6 -> RObjectPackFrame/7(CaptureMessage6)  "<RTICANMMCaptureMessage_6>"
  Bus Selector1/3 -> RObjectPackFrame/4(CaptureMessage3)  "<RTICANMMCaptureMessage_3>"
  Bus Selector1/5 -> RObjectPackFrame/6(CaptureMessage5)  "<RTICANMMCaptureMessage_5>"
  Bus Selector1/25 -> RObjectPackFrame/26(CaptureMessage25)  "<RTICANMMCaptureMessage_25>"
  Bus Selector1/15 -> RObjectPackFrame/16(CaptureMessage15)  "<RTICANMMCaptureMessage_15>"
  Bus Selector1/14 -> RObjectPackFrame/15(CaptureMessage14)  "<RTICANMMCaptureMessage_14>"
  Bus Selector1/16 -> RObjectPackFrame/17(CaptureMessage16)  "<RTICANMMCaptureMessage_16>"
  Bus Selector1/20 -> RObjectPackFrame/21(CaptureMessage20)  "<RTICANMMCaptureMessage_20>"
  Bus Selector1/19 -> RObjectPackFrame/20(CaptureMessage19)  "<RTICANMMCaptureMessage_19>"
  Bus Selector1/21 -> RObjectPackFrame/22(CaptureMessage21)  "<RTICANMMCaptureMessage_21>"
  Bus Selector1/24 -> RObjectPackFrame/25(CaptureMessage24)  "<RTICANMMCaptureMessage_24>"
  Bus Selector1/23 -> RObjectPackFrame/24(CaptureMessage23)  "<RTICANMMCaptureMessage_23>"
  Bus Selector1/17 -> RObjectPackFrame/18(CaptureMessage17)  "<RTICANMMCaptureMessage_17>"
  Bus Selector1/18 -> RObjectPackFrame/19(CaptureMessage18)  "<RTICANMMCaptureMessage_18>"
  Bus Selector1/22 -> RObjectPackFrame/23(CaptureMessage22)  "<RTICANMMCaptureMessage_22>"
  Bus Selector1/13 -> RObjectPackFrame/14(CaptureMessage13)  "<RTICANMMCaptureMessage_13>"
  Bus Selector1/9 -> RObjectPackFrame/10(CaptureMessage9)  "<RTICANMMCaptureMessage_9>"
  Bus Selector1/12 -> RObjectPackFrame/13(CaptureMessage12)  "<RTICANMMCaptureMessage_12>"
  Bus Selector1/11 -> RObjectPackFrame/12(CaptureMessage11)  "<RTICANMMCaptureMessage_11>"
  Bus Selector1/10 -> RObjectPackFrame/11(CaptureMessage10)  "<RTICANMMCaptureMessage_10>"
  Bus Selector1/8 -> RObjectPackFrame/9(CaptureMessage8)  "<RTICANMMCaptureMessage_8>"
  Bus Selector1/1 -> RObjectPackFrame/2(CaptureMessage1)  "<RTICANMMCaptureMessage_1>"
  Bus Selector1/2 -> RObjectPackFrame/3(CaptureMessage2)  "<RTICANMMCaptureMessage_2>"
  RObjectPackFrame/1(R_Objects_out) -> Bus Selector2/1
  Bus Selector2/1 -> [RObj_Status]  "<StatusFrame>"
  Bus Selector2/2 -> [RObj_Frames1]  "<Frames1>"
  Bus Selector2/3 -> [RObj_Frames2]  "<Frames2>"
  CAN2_Rx/1 -> Bus Selector1/1, Bus Selector/1
  [RObj_Status] -> RObj_Parser/1(RObj_Status)
  [RObj_Frames1] -> RObj_Parser/2(RObj_Frames1)
  [RObj_Frames2] -> RObj_Parser/3(RObj_Frames2)
  RObj_Parser/5(VHAL_SensorDefective_enum) -> VHAL_SensorDefective_enum/1
  RObj_Parser/1(VHAL_RadNofObjects_num) -> VHAL_RadNofObjects_num/1
  RObj_Parser/3(VHAL_SensorRxInvalid_enum) -> VHAL_SensorRxInvalid_enum/1
  RObj_Parser/7(VHAL_SensorSwitchedOff_enum) -> VHAL_SensorSwitchedOff_enum/1
  RObj_Parser/4(VHAL_SensorSupplyVoltage_V) -> VHAL_SensorSupplyVoltage_V/1
  RObj_Parser/6(VHAL_SensorMisaligned_enum) -> VHAL_SensorMisaligned_enum/1
  RObj_Parser/10(VHAL_LatDistToborderLeft_m) -> VHAL_LatDistToborderLeft_m/1
  RObj_Parser/2(VHAL_MeasCounter_num) -> VHAL_MeasCounter_num/1
  RObj_Parser/8(VHAL_SensorExternalDisturbed_enum) -> VHAL_SensorExternalDisturbed_enum/1
  RObj_Parser/9(VHAL_SensorOutputReduced_enum) -> VHAL_SensorOutputReduced_enum/1
  RObj_Parser/11(VHAL_LatDistToborderRight_m) -> VHAL_LatDistToborderRight_m/1
  RObj_Parser/12(VHAL_RadObjRolCountVect40_num) -> VHAL_RadObjRolCountVect40_num/1
  RObj_Parser/13(VHAL_RadObjIDVect40_num) -> VHAL_RadObjIDVect40_num/1
  RObj_Parser/14(VHAL_RadObjXDisplVect40_m) -> VHAL_RadObjXDisplVect40_m/1
  RObj_Parser/15(VHAL_RadObjVrelXVect40_mps) -> VHAL_RadObjVrelXVect40_mps/1
  RObj_Parser/16(VHAL_RadObjAccelXVect40_mps2) -> VHAL_RadObjAccelXVect40_mps2/1
  RObj_Parser/17(VHAL_RadObjYDisplVect40_m) -> VHAL_RadObjYDisplVect40_m/1
  RObj_Parser/18(VHAL_RadObjDynPropVect40_enum) -> VHAL_RadObjDynPropVect40_enum/1
  RObj_Parser/19(VHAL_RadObjPExistVect40_enum) -> VHAL_RadObjPExistVect40_enum/1
  RObj_Parser/20(VHAL_RadObjMeasStatVect40_enum) -> VHAL_RadObjMeasStatVect40_enum/1
  RObj_Parser/21(VHAL_RadObjWidthVect40_m) -> VHAL_RadObjWidthVect40_m/1
  RObj_Parser/22(VHAL_RadObjLengthVect40_m) -> VHAL_RadObjLengthVect40_m/1
  RObj_Parser/23(VHAL_RadObjRCSVect40_num) -> VHAL_RadObjRCSVect40_num/1
  RObj_Parser/24(VHAL_RadObjVrelYVect40_mps) -> VHAL_RadObjVrelYVect40_mps/1
  RObj_Parser/25(VHAL_RadObjProbVect40_num) -> VHAL_RadObjProbVect40_num/1
  RObj_Parser/26(VHAL_RadWarningLevel_enum) -> VHAL_RadWarningLevel_enum/1
  RObj_Parser/27(VHAL_RadWarningObjID_num) -> VHAL_RadWarningObjID_num/1

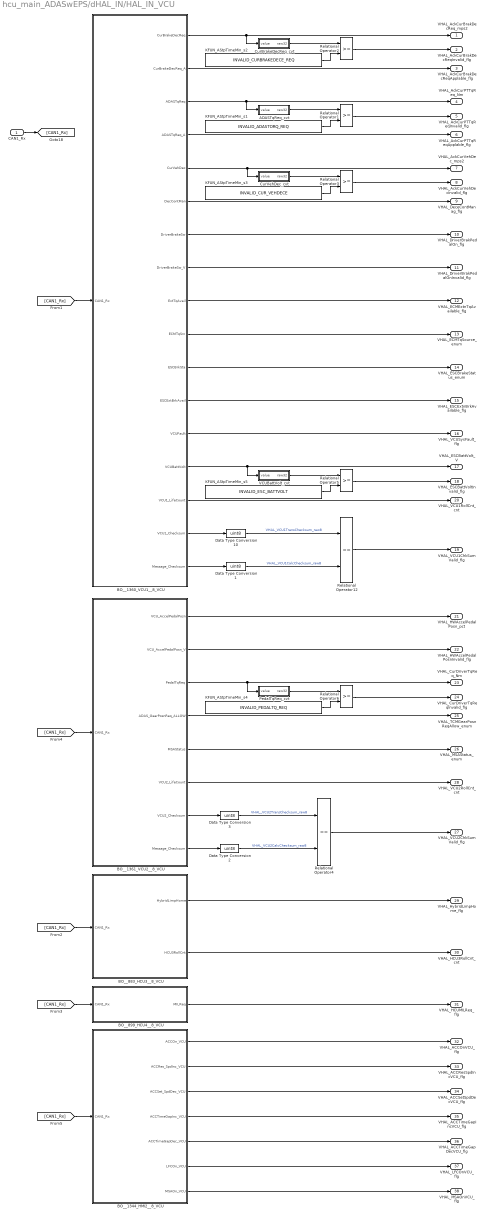
== system hcu_main_ADASwEPS/dHAL_IN/HAL_IN_VCU ==
  CAN1_Rx : Inport
  ADASTqReq_cvt : Subsystem  mask(ConvertOut){gain=0.2, offset=-100}
      mask help:
      | Conversion Formula
      |
      | The conversion formula is
      |
      | raw_value = (physical_value - Offset) / Factor
      |
      | where physical_value is the value of the signal after it is saturated using the specified Min and Max values. raw_value is the packed signal value.
  BO__1344_HMI2__8_VCU : Subsystem
  BO__1360_VCU1__8_VCU : Subsystem
  BO__1361_VCU2__8_VCU : Subsystem
  BO__883_HCU3__8_VCU : Subsystem
  BO__899_HCU4__8_VCU : Subsystem
  CurBrakeDecReq_cvt : Subsystem  mask(ConvertOut){gain=0.1, offset=0}
      mask help:
      | Conversion Formula
      |
      | The conversion formula is
      |
      | raw_value = (physical_value - Offset) / Factor
      |
      | where physical_value is the value of the signal after it is saturated using the specified Min and Max values. raw_value is the packed signal value.
  CurVehDec_cvt : Subsystem  mask(ConvertOut){gain=0.1, offset=0}
      mask help:
      | Conversion Formula
      |
      | The conversion formula is
      |
      | raw_value = (physical_value - Offset) / Factor
      |
      | where physical_value is the value of the signal after it is saturated using the specified Min and Max values. raw_value is the packed signal value.
  Data Type Conversion{1..3,10} (4 alike) : DataTypeConversion  OutDataTypeStr=uint8
  KFUN_AStpTimeMin_s1 : Constant  Value=INVALID_ADASTORQ_REQ
  KFUN_AStpTimeMin_s2 : Constant  Value=INVALID_CURBRAKEDECE_REQ
  KFUN_AStpTimeMin_s3 : Constant  Value=INVALID_CUR_VEHDECE
  KFUN_AStpTimeMin_s4 : Constant  Value=INVALID_PEDALTQ_REQ
  KFUN_AStpTimeMin_s5 : Constant  Value=INVALID_ESC_BATTVOLT
  PedalTqReq_cvt : Subsystem  mask(ConvertOut){gain=0.2, offset=-100}
      mask help:
      | Conversion Formula
      |
      | The conversion formula is
      |
      | raw_value = (physical_value - Offset) / Factor
      |
      | where physical_value is the value of the signal after it is saturated using the specified Min and Max values. raw_value is the packed signal value.
  Relational Operator{1..3,5..6} (5 alike) : RelationalOperator  OutDataTypeStr=boolean
  Relational Operator12 : RelationalOperator  Operator===  OutDataTypeStr=boolean
  Relational Operator4 : RelationalOperator  Operator===  OutDataTypeStr=boolean
  VCUBattVolt_cvt : Subsystem  mask(ConvertOut){gain=0.1, offset=0}
      mask help:
      | Conversion Formula
      |
      | The conversion formula is
      |
      | raw_value = (physical_value - Offset) / Factor
      |
      | where physical_value is the value of the signal after it is saturated using the specified Min and Max values. raw_value is the packed signal value.
  VHAL_AckCurBrakDecReq_mps2 : Outport
  VHAL_AckCurBrakDecReqInvalid_flg : Outport  Port=2
  VHAL_AckCurBrakDecReqApplable_flg : Outport  Port=3
  VHAL_AckCurPTTqReq_Nm : Outport  Port=4
  VHAL_AckCurPTTqReqInvalid_flg : Outport  Port=5
  VHAL_AckCurPTTqReqApplable_flg : Outport  Port=6
  VHAL_AckCurVehDec_mps2 : Outport  Port=7
  VHAL_AckCurVehDecInvalid_flg : Outport  Port=8
  VHAL_DeceContManag_flg : Outport  Port=9
  VHAL_DriverBrakPedalOn_flg : Outport  Port=10
  VHAL_DriverBrakPedalOnInvalid_flg : Outport  Port=11
  VHAL_ECMExtnTqAvailable_flg : Outport  Port=12
  VHAL_ECMTqSource_enum : Outport  Port=13
  VHAL_ESCBrakeStatus_enum : Outport  Port=14
  VHAL_ESCExtnBrkAvailable_flg : Outport  Port=15
  VHAL_VCUSysFault_flg : Outport  Port=16
  VHAL_ESCBattVolt_V : Outport  Port=17
  VHAL_ESCBattVoltInvalid_flg : Outport  Port=18
  VHAL_VCU1ChkSumValid_flg : Outport  Port=19
  VHAL_VCU1RollCnt_cnt : Outport  Port=20
  VHAL_HWAccelPedalPosn_pct : Outport  Port=21
  VHAL_HWAccelPedalPosnInvalid_flg : Outport  Port=22
  VHAL_CurDriverTqReq_Nm : Outport  Port=23
  VHAL_CurDriverTqReqInvalid_flg : Outport  Port=24
  VHAL_TCMGearPosnReqAllow_enum : Outport  Port=25
  VHAL_MSAStatus_enum : Outport  Port=26
  VHAL_VCU2ChkSumValid_flg : Outport  Port=27
  VHAL_VCU2RollCnt_cnt : Outport  Port=28
  VHAL_HybridLimpHome_flg : Outport  Port=29
  VHAL_HCU3RollCnt_cnt : Outport  Port=30
  VHAL_HCUMILReq_flg : Outport  Port=31
  VHAL_ACCOnVCU_flg : Outport  Port=32
  VHAL_ACCResSpdIncVCU_flg : Outport  Port=33
  VHAL_ACCSetSpdDecVCU_flg : Outport  Port=34
  VHAL_ACCTimeGapIncVCU_flg : Outport  Port=35
  VHAL_ACCTimeGapDecVCU_flg : Outport  Port=36
  VHAL_LFCOnVCU_flg : Outport  Port=37
  VHAL_MSAOnVCU_flg : Outport  Port=38
  wires:
  [CAN1_Rx] -> BO__1344_HMI2__8_VCU/1(CAN1_Rx)
  BO__1344_HMI2__8_VCU/6(LFCOn_VCU) -> VHAL_LFCOnVCU_flg/1
  BO__1344_HMI2__8_VCU/4(ACCTimeGapInc_VCU) -> VHAL_ACCTimeGapIncVCU_flg/1
  BO__1344_HMI2__8_VCU/5(ACCTimeGapDec_VCU) -> VHAL_ACCTimeGapDecVCU_flg/1
  BO__1344_HMI2__8_VCU/3(ACCSet_SpdDec_VCU) -> VHAL_ACCSetSpdDecVCU_flg/1
  BO__1344_HMI2__8_VCU/2(ACCRes_SpdInc_VCU) -> VHAL_ACCResSpdIncVCU_flg/1
  BO__1344_HMI2__8_VCU/1(ACCOn_VCU) -> VHAL_ACCOnVCU_flg/1
  BO__1360_VCU1__8_VCU/2(CurBrakeDecReq_A) -> VHAL_AckCurBrakDecReqApplable_flg/1
  BO__1360_VCU1__8_VCU/4(ADASTqReq_A) -> VHAL_AckCurPTTqReqApplable_flg/1
  Relational Operator3/1 -> VHAL_AckCurVehDecInvalid_flg/1
  BO__1360_VCU1__8_VCU/6(DecContMan) -> VHAL_DeceContManag_flg/1
  BO__1360_VCU1__8_VCU/7(DriverBrakeSw) -> VHAL_DriverBrakPedalOn_flg/1
  BO__1360_VCU1__8_VCU/9(ExtTqAvail) -> VHAL_ECMExtnTqAvailable_flg/1
  BO__1360_VCU1__8_VCU/10(ECMTqSrc) -> VHAL_ECMTqSource_enum/1
  BO__1360_VCU1__8_VCU/11(ESCBrkSta) -> VHAL_ESCBrakeStatus_enum/1
  BO__1360_VCU1__8_VCU/12(ESCExtBrkAvail) -> VHAL_ESCExtnBrkAvailable_flg/1
  BO__1360_VCU1__8_VCU/13(VCUFault) -> VHAL_VCUSysFault_flg/1
  Relational Operator12/1 -> VHAL_VCU1ChkSumValid_flg/1
  BO__1360_VCU1__8_VCU/15(VCU1_LifeCount) -> VHAL_VCU1RollCnt_cnt/1
  BO__883_HCU3__8_VCU/1(HybridLimpHome) -> VHAL_HybridLimpHome_flg/1
  BO__883_HCU3__8_VCU/2(HCU3RollCnt) -> VHAL_HCU3RollCnt_cnt/1
  BO__899_HCU4__8_VCU/1(MILReq) -> VHAL_HCUMILReq_flg/1
  CAN1_Rx/1 -> [CAN1_Rx]
  [CAN1_Rx] -> BO__1360_VCU1__8_VCU/1(CAN1_Rx)
  [CAN1_Rx] -> BO__883_HCU3__8_VCU/1(CAN1_Rx)
  [CAN1_Rx] -> BO__899_HCU4__8_VCU/1(CAN1_Rx)
  Data Type Conversion10/1 -> Relational Operator12/1  "VHAL_VCU1TransChecksum_raw8"
  Data Type Conversion1/1 -> Relational Operator12/2  "VHAL_VCU1CalcChecksum_raw8"
  BO__1360_VCU1__8_VCU/16(VCU1_Checksum) -> Data Type Conversion10/1
  BO__1360_VCU1__8_VCU/17(Message_Checksum) -> Data Type Conversion1/1
  [CAN1_Rx] -> BO__1361_VCU2__8_VCU/1(CAN1_Rx)
  Relational Operator4/1 -> VHAL_VCU2ChkSumValid_flg/1
  Data Type Conversion3/1 -> Relational Operator4/1  "VHAL_VCU2TransChecksum_raw8"
  Data Type Conversion2/1 -> Relational Operator4/2  "VHAL_VCU2CalcChecksum_raw8"
  BO__1361_VCU2__8_VCU/7(VCU2_Checksum) -> Data Type Conversion3/1
  BO__1361_VCU2__8_VCU/8(Message_Checksum) -> Data Type Conversion2/1
  BO__1361_VCU2__8_VCU/1(VCU_AccelPedalPosn) -> VHAL_HWAccelPedalPosn_pct/1
  BO__1361_VCU2__8_VCU/2(VCU_AccelPedalPosn_V) -> VHAL_HWAccelPedalPosnInvalid_flg/1
  BO__1361_VCU2__8_VCU/6(VCU2_LifeCount) -> VHAL_VCU2RollCnt_cnt/1
  BO__1344_HMI2__8_VCU/7(MSAOn_VCU) -> VHAL_MSAOnVCU_flg/1
  BO__1360_VCU1__8_VCU/1(CurBrakeDecReq) -> CurBrakeDecReq_cvt/1(value), VHAL_AckCurBrakDecReq_mps2/1
  KFUN_AStpTimeMin_s2/1 -> Relational Operator2/2
  CurBrakeDecReq_cvt/1(raw32) -> Relational Operator2/1
  Relational Operator2/1 -> VHAL_AckCurBrakDecReqInvalid_flg/1
  BO__1360_VCU1__8_VCU/3(ADASTqReq) -> ADASTqReq_cvt/1(value), VHAL_AckCurPTTqReq_Nm/1
  KFUN_AStpTimeMin_s1/1 -> Relational Operator1/2
  ADASTqReq_cvt/1(raw32) -> Relational Operator1/1
  Relational Operator1/1 -> VHAL_AckCurPTTqReqInvalid_flg/1
  BO__1360_VCU1__8_VCU/5(CurVehDec) -> CurVehDec_cvt/1(value), VHAL_AckCurVehDec_mps2/1
  KFUN_AStpTimeMin_s3/1 -> Relational Operator3/2
  CurVehDec_cvt/1(raw32) -> Relational Operator3/1
  BO__1360_VCU1__8_VCU/14(VCUBattVolt) -> VCUBattVolt_cvt/1(value), VHAL_ESCBattVolt_V/1
  KFUN_AStpTimeMin_s5/1 -> Relational Operator5/2
  VCUBattVolt_cvt/1(raw32) -> Relational Operator5/1
  Relational Operator5/1 -> VHAL_ESCBattVoltInvalid_flg/1
  BO__1361_VCU2__8_VCU/4(ADAS_GearPosnReq_ALLOW) -> VHAL_TCMGearPosnReqAllow_enum/1
  BO__1361_VCU2__8_VCU/5(MSAStatus) -> VHAL_MSAStatus_enum/1
  Relational Operator6/1 -> VHAL_CurDriverTqReqInvalid_flg/1
  BO__1361_VCU2__8_VCU/3(PedalTqReq) -> PedalTqReq_cvt/1(value), VHAL_CurDriverTqReq_Nm/1
  KFUN_AStpTimeMin_s4/1 -> Relational Operator6/2
  PedalTqReq_cvt/1(raw32) -> Relational Operator6/1
  BO__1360_VCU1__8_VCU/8(DriverBrakeSw_V) -> VHAL_DriverBrakPedalOnInvalid_flg/1
